simulink model "functionModel"  (R2015b)
settings: Solver=FixedStepAuto  StartTime=0.0  StopTime=inf  FixedStep=0.01  RelTol=1e-1
undefined symbols (not defined in the file or in its folder): CFuzzymin
libraries: fuzblock x1
settings Model: Creator=Pepe  LastModifiedBy=Pepe
settings SolverCC: MaxConsecutiveMinStep=10  ZeroCrossAlgorithm=Adaptive

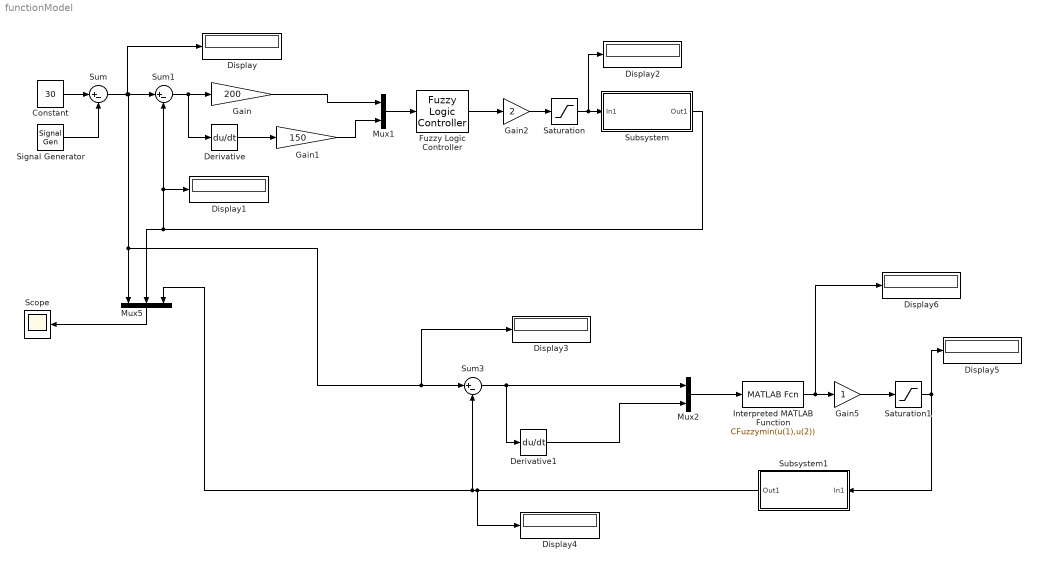
== system functionModel ==
  Constant : Constant  Value=30
  Derivative : Derivative
  Derivative1 : Derivative
  Display{,1..6} (7 alike) : Display
  Fuzzy Logic Controller : fuzblock/Fuzzy Logic  Controller  fis=P1
  Gain : Gain  Gain=200
  Gain1 : Gain  Gain=150
  Gain2 : Gain  Gain=2
  Gain5 : Gain
  Interpreted MATLAB Function : MATLABFcn  MATLABFcn=CFuzzymin(u(1),u(2))
  Mux1 : Mux  Inputs=2
  Mux2 : Mux  Inputs=2
  Mux5 : Mux  Inputs=3
  Saturation : Saturate  UpperLimit=5  LowerLimit=0
  Saturation1 : Saturate  UpperLimit=2  LowerLimit=0
  Scope : Scope
  Signal Generator : SignalGenerator  WaveForm=square  Amplitude=10  Frequency=0.002
  Subsystem : Subsystem
  Subsystem1 : Subsystem
  Sum : Sum  Inputs=|+-
  Sum1 : Sum  Inputs=|+-
  Sum3 : Sum  Inputs=|+-
  wires:
  Constant/1 -> Sum/1
  Signal Generator/1 -> Sum/2
  Sum1/1 -> Gain/1, Derivative/1
  Derivative/1 -> Gain1/1
  Gain/1 -> Mux1/1
  Gain1/1 -> Mux1/2
  Mux1/1 -> Fuzzy Logic Controller/1
  Fuzzy Logic Controller/1 -> Gain2/1
  Subsystem/1(Out1) -> Mux5/2, Display1/1, Sum1/2
  Gain2/1 -> Saturation/1
  Saturation/1 -> Display2/1, Subsystem/1(In1)
  Mux5/1 -> Scope/1
  Sum3/1 -> Derivative1/1, Mux2/1
  Gain5/1 -> Saturation1/1
  Saturation1/1 -> Subsystem1/1(In1), Display5/1
  Sum/1 -> Display3/1, Sum3/1, Mux5/1, Sum1/1, Display/1
  Interpreted MATLAB Function/1 -> Display6/1, Gain5/1
  Mux2/1 -> Interpreted MATLAB Function/1
  Subsystem1/1(Out1) -> Display4/1, Mux5/3, Sum3/2
  Derivative1/1 -> Mux2/2

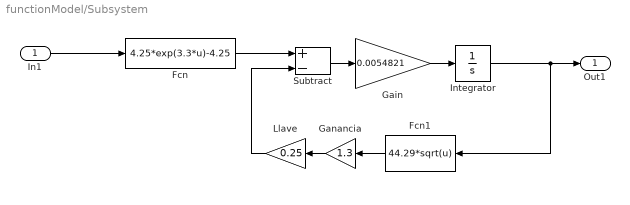
== system functionModel/Subsystem ==
  In1 : Inport
  Fcn : Fcn  Expr=4.25*exp(3.3*u)-4.25
  Fcn1 : Fcn  Expr=44.29*sqrt(u)
  Gain : Gain  Gain=0.0054821
  Ganancia : Gain  Gain=1.3
  Integrator : Integrator  InitialCondition=15  LimitOutput=on  UpperSaturationLimit=78  LowerSaturationLimit=0
  Llave : Gain  Gain=0.25
  Subtract : Sum  Inputs=+-
  Out1 : Outport
  wires:
  Llave/1 -> Subtract/2
  Fcn1/1 -> Ganancia/1
  Gain/1 -> Integrator/1
  Fcn/1 -> Subtract/1
  Ganancia/1 -> Llave/1
  Subtract/1 -> Gain/1
  Integrator/1 -> Out1/1, Fcn1/1
  In1/1 -> Fcn/1

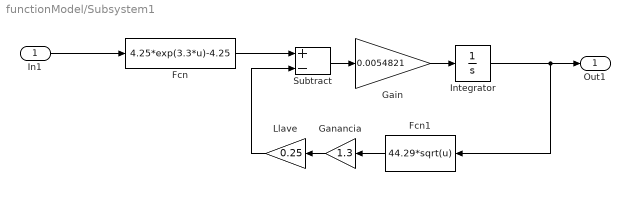
== system functionModel/Subsystem1 ==
  In1 : Inport
  Fcn : Fcn  Expr=4.25*exp(3.3*u)-4.25
  Fcn1 : Fcn  Expr=44.29*sqrt(u)
  Gain : Gain  Gain=0.0054821
  Ganancia : Gain  Gain=1.3
  Integrator : Integrator  InitialCondition=15  LimitOutput=on  UpperSaturationLimit=78  LowerSaturationLimit=0
  Llave : Gain  Gain=0.25
  Subtract : Sum  Inputs=+-
  Out1 : Outport
  wires:
  Llave/1 -> Subtract/2
  Fcn1/1 -> Ganancia/1
  Gain/1 -> Integrator/1
  Fcn/1 -> Subtract/1
  Ganancia/1 -> Llave/1
  Subtract/1 -> Gain/1
  Integrator/1 -> Out1/1, Fcn1/1
  In1/1 -> Fcn/1
